simulink model "L1_Fxx_Spurmittenfuehrung"  (R2021a)
settings: Solver=ode45  StartTime=0.0  StopTime=10.0  RelTol=1e-3  EnableMultiTasking=on
PostLoadFcn:
  | s = find_system('Name','Reglerverstärkung')
  | set_param(s{1},'Gain','0.005')
  | s = find_system('Name','Wetter / Weather')
  | set_param(s{1},'After','0%-0.01')
InitFcn:
  | %params
  | w=3;
  | D=0.6;
  | v=80/3.6;
  | vch=30;
  | n=113;
StopFcn:
  | figure(n);clf;
  | sc= get(0,'screensize')
  | h = gcf;
  | h.Position = [sc(4)/2,sc(4)/10,sc(3)/3.5,sc(4)/1.3];
  | %h.Position(4) = h.Position(4)*1.5;
  | 
  | subplot(2,1,1)
  | 
  | hold on; box on; grid on;
  | vv=v;
  | vv = 1; % DO
  | s1 = logsout.getElement('y_Strasse').Values;
  | s2 = logsout.getElement('y_Fzg').Values;
  | s3 = logsout.getElement('y_Soll').Values;
  | 
  | l1 = plot(s2.Time*vv,s1.Data,'Color',0.5*[1,1,1]);
  | l2 = plot(s1.Time*vv,s2.Data,'m:');
  | 
  | ylabel('y - Coordinate [m]','FontSize',16)
  | 
  | l1.LineWidth=4;
  | l2.LineWidth=2;
  | 
  | %xlim([0,10])
  | grid on;
  | 
  | %a=gca;
  | %a.DataAspectRatio = [1 1 1];
  | legend('Street','Car Position','Location','northwest','FontSize',16)
  | 
  | %%%%%%%%%%%%%%%%%%%%%%%%%%%%%%%%%%%%
  | subplot(2,1,2)
  | hold on; box on; grid on;
  | 
  | l3 = plot(s3.Time,s3.Data-s2.Data+s1.Data);
  | %l4 = plot(s3.Time,s3.Data);
  | 
  | legend('Control Error','Location','northwest','FontSize',16)
  | l3.LineWidth=2;
  | %l4.LineWidth=2;
  | 
  | xlabel('Time [s]','FontSize',16)
  | ylabel('Error [m]','FontSize',16)
  | 
  | 
  | figure(n);
undefined symbols (not defined in the file or in its folder): sigbuilder_block
settings Model: Creator=Nitzsche  LastModifiedBy=Ossmann
settings SolverCC: AlgebraicLoopSolver=TrustRegion
settings DataIOCC: LimitDataPoints=on  ReturnWorkspaceOutputs=off
settings OptimizationCC: LifeSpan=inf
settings DebuggingCC: AllowSymbolicDim=off  SFUnexpectedBacktrackingDiag=warning  SFNoUnconditionalDefaultTransitionDiag=warning  SFExecutionAtInitializationDiag=none  SFMachineParentedDataDiag=warning  ArithmeticOperatorsInVariantConditions=warning
settings ModelReferenceCC: PropagateSignalLabelsOutOfModel=off
settings SFSimCC: SimUseLocalCustomCode=off  CustomCodeUndefinedFunction=UseInterfaceOnly
settings RTWCC: RTWUseLocalCustomCode=off
settings CodeAppCC: StateflowObjectComments=on
settings GRTTargetCC: TargetLangStandard=C89/C90 (ANSI)
settings ConfigComp: CovMetricSettings=dw  CovSaveCumulativeToWorkspaceVar=on  CovSaveSingleToWorkspaceVar=on  CovExternalEMLEnable=off

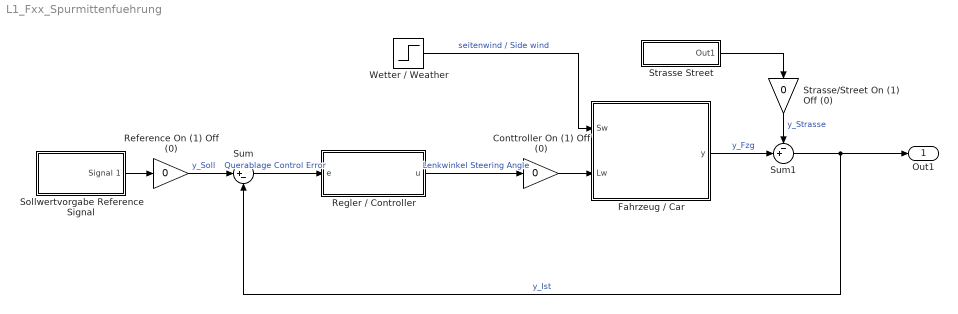
== system L1_Fxx_Spurmittenfuehrung ==
  Conttroller On (1) Off (0) : Gain  Gain=0
  Fahrzeug / Car : Subsystem
  Reference On (1) Off (0) : Gain  Gain=0
  "Regler / Controller " : Subsystem
  Sollwertvorgabe Reference Signal : Subsystem  Tag=STV Subsys  LoadFcn=sigbuilder_block('load');  StartFcn=sigbuilder_block('start');  StopFcn=sigbuilder_block('stop');  ClipboardFcn=sigbuilder_block('clipboard');  mask(Sigbuilder block){tuvar=[0:10]}
      mask help: Simulink:masks:SigbuilderBlock_MD
      mask init:
      | if ~strcmp(get_param(bdroot(gcbh),'SimulationStatus'),'stopped') tuvar = sigbuilder_block('maskInit'); end
      settings: CopyFcn=sigbuilder_block('copy');  DeleteFcn=sigbuilder_block('delete');  ModelCloseFcn=sigbuilder_block('modelClose');  PreSaveFcn=sigbuilder_block('preSave');  PauseFcn=sigbuilder_block('pause');  ContinueFcn=sigbuilder_block('continue');  NameChangeFcn=sigbuilder_block('namechange');  OpenFcn=sigbuilder_block('open',[117 225.6 550.5 360.6 ]);  CloseFcn=sigbuilder_block('close');
      mask Display: plot(0, 0, 100, 100,[2, 2, 32, 32, 2], [68, 8, 8, 68, 68],[32, 2], [38, 38], [32, 19, 2],[53, 60, 44], [32, 17, 17, 2],[16, 16, 31, 31]);txt = getActiveGroup(gcbh);text(2, 100, txt,'verticalAlignment', 'top');
  "Strasse Street " : Subsystem
  Strasse/Street On (1) Off (0) : Gain  Gain=0
  Sum : Sum  Inputs=|+-
  Sum1 : Sum  Inputs=-+|
  Wetter / Weather : Step  Time=3  After=0%-0.01  SampleTime=0
  Out1 : Outport  VectorParamsAs1DForOutWhenUnconnected=off
  wires:
  Sollwertvorgabe Reference Signal/1(Signal 1) -> Reference On (1) Off (0)/1
  Sum/1 -> "Regler / Controller "/1(e)  "Querablage Control Error"
  "Regler / Controller "/1(u) -> Conttroller On (1) Off (0)/1  "Lenkwinkel Steering Angle"
  Wetter / Weather/1 -> Fahrzeug / Car/1(Sw)  "seitenwind / Side wind"
  Fahrzeug / Car/1(y) -> Sum1/2  "y_Fzg"
  Sum1/1 -> Sum/2, Out1/1  "y_Ist"
  "Strasse Street "/1(Out1) -> Strasse/Street On (1) Off (0)/1
  Strasse/Street On (1) Off (0)/1 -> Sum1/1  "y_Strasse"
  Reference On (1) Off (0)/1 -> Sum/1  "y_Soll"
  Conttroller On (1) Off (0)/1 -> Fahrzeug / Car/2(Lw)

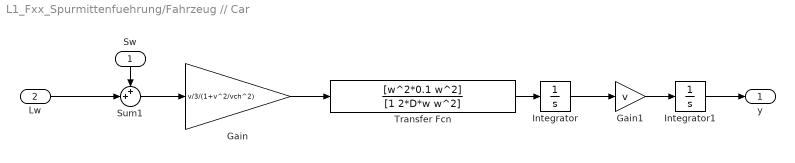
== system L1_Fxx_Spurmittenfuehrung/Fahrzeug // Car ==
  Sw : Inport
  Lw : Inport  Port=2
  Gain : Gain  Gain=v/3/(1+v^2/vch^2)
  Gain1 : Gain  Gain=v
  Integrator : Integrator
  Integrator1 : Integrator
  Sum1 : Sum  Inputs=++|
  Transfer Fcn : TransferFcn  Numerator=[w^2*0.1 w^2]  Denominator=[1 2*D*w w^2]
  y : Outport  VectorParamsAs1DForOutWhenUnconnected=off
  wires:
  Sum1/1 -> Gain/1
  Gain1/1 -> Integrator1/1
  Integrator/1 -> Gain1/1
  Transfer Fcn/1 -> Integrator/1
  Lw/1 -> Sum1/2
  Gain/1 -> Transfer Fcn/1
  Sw/1 -> Sum1/1
  Integrator1/1 -> y/1

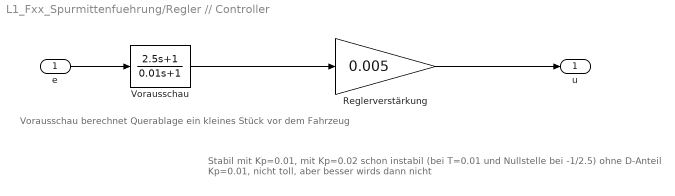
== system L1_Fxx_Spurmittenfuehrung/Regler // Controller  ==
  note: Vorausschau berechnet Querablage ein kleines Stück vor dem Fahrzeug
  note: Stabil mit Kp=0.01, mit Kp=0.02 schon instabil (bei T=0.01 und Nullstelle bei -1/2.5) ohne D-Anteil Kp=0.01, nicht toll, aber besser wirds dann nicht
  e : Inport
  Reglerverstärkung : Gain  Gain=0.005
  Vorausschau : TransferFcn  Numerator=[2.5 1]  Denominator=[0.01 1]
  u : Outport  VectorParamsAs1DForOutWhenUnconnected=off
  wires:
  e/1 -> Vorausschau/1
  Vorausschau/1 -> Reglerverstärkung/1
  Reglerverstärkung/1 -> u/1

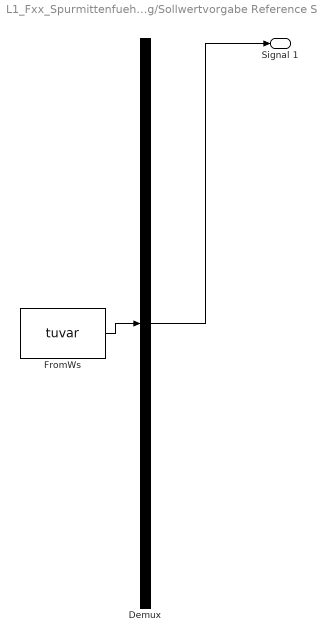
== system L1_Fxx_Spurmittenfuehrung/Sollwertvorgabe Reference Signal ==
  Demux : Demux  Tag=STV Demux  Outputs=1
      settings: DisplayOption=none
  FromWs : FromWorkspace  Tag=STV FromWs  VariableName=tuvar
      SigBuilderData=|
      | common.afterFinalStr = 'Extrapolate'
      | common.sampleTime = 0
      | dataSet.timeRange = [0 10]
      | dataSet.name = 'Group 1'
      | sbobj.Groups.Name = 'Group 1'
      | sbobj.Groups.Signals.Name = 'Signal 1'
      | sbobj.Groups.Signals.XData = [0 1.02 5 10]
      | sbobj.Groups.Signals.YData = [0 0 0.4 0.4]
  Signal 1 : Outport  Tag=STV Outport  VectorParamsAs1DForOutWhenUnconnected=off
  wires:
  Demux/1 -> Signal 1/1
  FromWs/1 -> Demux/1

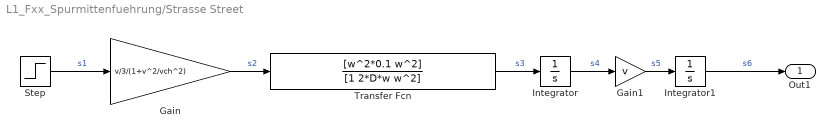
== system L1_Fxx_Spurmittenfuehrung/Strasse Street  ==
  Gain : Gain  Gain=v/3/(1+v^2/vch^2)
  Gain1 : Gain  Gain=v
  Integrator : Integrator
  Integrator1 : Integrator
  Step : Step  Time=0.5  After=0.012  SampleTime=0
  Transfer Fcn : TransferFcn  Numerator=[w^2*0.1 w^2]  Denominator=[1 2*D*w w^2]
  Out1 : Outport  VectorParamsAs1DForOutWhenUnconnected=off
  wires:
  Step/1 -> Gain/1  "s1"
  Transfer Fcn/1 -> Integrator/1  "s3"
  Integrator1/1 -> Out1/1  "s6"
  Integrator/1 -> Gain1/1  "s4"
  Gain1/1 -> Integrator1/1  "s5"
  Gain/1 -> Transfer Fcn/1  "s2"
